simulink model "Linm_doubl_int"  (Simulink 7.5)
settings: Solver=ode45  StartTime=0.0  StopTime=10.0  RelTol=1e-3
settings Model: Creator=fclaveau  LastModifiedBy=fclaveau

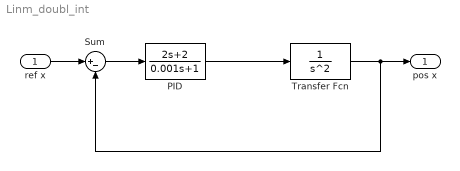
== system Linm_doubl_int ==
  ref x : Inport
  PID : TransferFcn  Numerator=[2 2]  Denominator=[0.001 1]
  Sum : Sum  Inputs=|+-  OutDataType=fixdt(1, 16)  OutScaling=2^0
  Transfer Fcn : TransferFcn  Denominator=[1 0 0]
  pos x : Outport
  wires:
  Sum/1 -> PID/1
  ref x/1 -> Sum/1
  PID/1 -> Transfer Fcn/1
  Transfer Fcn/1 -> pos x/1, Sum/2
